simulink model "PMSMvelocityController"  (R2013b)
settings: Solver=FixedStepDiscrete  StartTime=0.0  StopTime=inf  RelTol=1e-3
values from neighbouring files (symbols this model uses):
  ctrlConst = struct    [applicationData.m]
  paramCurrentI = createParameter(      20000,      [0 25000],      DT_PRECISION_LO,      'Volt/Ampere',     'I gain parameter in Currrent Control PI Controller')    [applicationData.m]
  paramCurrentP = createParameter(     10,     [0 100],     DT_PRECISION_LO,     'Volt/Ampere',     'P gain parameter in Current Control PI Controller')    [applicationData.m]
  paramCurrentPIVoltageSat = createParameter(     0.9 * (ctrlConst.VoltageMax/2),     [0 (ctrlConst.VoltageMax/2)],     DT_PRECISION_LO,     'Volt',     'Maximum voltage command output from current controller')    [applicationData.m]
  paramVelocityI = createParameter(      0.275,      [0 2],      DT_PRECISION_LO,      'Ampere/(rad/sec)',     'I gain parameter in Velocity Control PI Controller')    [applicationData.m]
  paramVelocityP = createParameter(     0.2814,     [0 1],     DT_PRECISION_LO,     'Ampere/(rad/sec)',     'P gain parameter in Velocity Control PI Controller')    [applicationData.m]
  paramVelocityPICurrentSat = createParameter(     2,     [0 6],     DT_PRECISION_LO,     'Ampere',     'Maximum Current Command Output from Velocity Controller')    [applicationData.m]
libraries: simulink x11, libDataType x3, libAbcDqFixpt x2, libSinCosFixpt x1, libSinCosFixptC2000 x1, libSinCos x1
settings Model: SimulationMode=accelerator  Creator=mcorless  LastModifiedBy=rchladny
settings DataIOCC: SaveOutput=off  SaveTime=off
settings OptimizationCC: InlineParams=on  UseSpecifiedMinMax=on  ZeroExternalMemoryAtStartup=off  NoFixptDivByZeroProtection=on  EfficientFloat2IntCast=on  OptimizeModelRefInitCode=on  LifeSpan=1
settings DebuggingCC: InheritedTsInSrcMsg=none  ParameterPrecisionLossMsg=none  ModelReferenceSymbolNameMessage=none  StateNameClashWarn=warning
settings HardwareCC: ProdBitPerChar=16  ProdBitPerInt=16  ProdBitPerPointer=16  ProdLargestAtomicInteger=Integer  ProdIntDivRoundTo=Zero  ProdEndianess=LittleEndian  ProdWordSize=16  ProdHWDeviceType=Texas Instruments->C2000
settings ModelReferenceCC: ModelReferenceNumInstancesAllowed=Single
settings RTWCC: SystemTargetFile=ert.tlc  TemplateMakefile=ec_target.tmf  Description=Embedded Coder  GenerateReport=on  ProcessScript=ert_make_rtw_hook  IncludeHyperlinkInReport=on  LaunchReport=on  PortableWordSizes=on  GenerateTraceInfo=on  GenerateTraceReport=on  GenerateTraceReportSl=on  GenerateTraceReportSf=on  GenerateTraceReportEml=on  GenerateCodeMetricsReport=on  RTWCompilerOptimization=On
settings CodeAppCC: IgnoreCustomStorageClasses=off
settings ERTTargetCC: CodeReplacementLibrary=C89/C90 (ANSI)  GenerateSampleERTMain=on  IncludeMdlTerminateFcn=off  CombineSignalStateStructs=on  SuppressErrorStatus=on  ERTCustomFileTemplate=example_file_process.tlc  ERTFilePackagingFormat=Compact  SuppressUnreachableDefaultCases=on

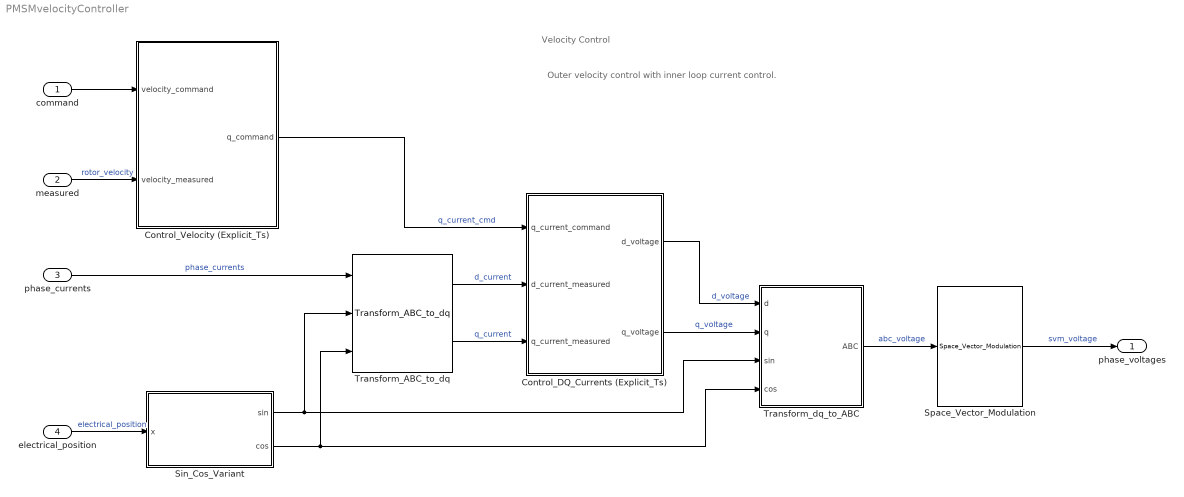
== system PMSMvelocityController ==
  note: Outer velocity control with inner loop current control.
  note: Velocity Control
  command : Inport  OutMin=-ctrlConst.VelocityMax  OutMax=ctrlConst.VelocityMax  OutDataTypeStr=DT_PRECISION_LO  PortDimensions=1  SampleTime=ctrlConst.TsControlLawPort  Interpolate=off
      settings: AttributesFormatString=-------------------\nMin = %<OutMin>\nMax = %<OutMax>
  measured : Inport  Port=2  OutMin=-ctrlConst.VelocityMax  OutMax=ctrlConst.VelocityMax  OutDataTypeStr=DT_PRECISION_LO  PortDimensions=1
      settings: AttributesFormatString=-------------------\nMin = %<OutMin>\nMax = %<OutMax>
  phase_currents : Inport  Port=3  OutMin=-ctrlConst.CurrentMax  OutMax=ctrlConst.CurrentMax  OutDataTypeStr=DT_PRECISION_LO  PortDimensions=2  Interpolate=off
      settings: AttributesFormatString=-------------------\nMin = %<OutMin>\nMax = %<OutMax>
  electrical_position : Inport  Port=4  OutMin=0  OutMax=2*pi  OutDataTypeStr=DT_PRECISION_LO  PortDimensions=1  Interpolate=off
      settings: AttributesFormatString=-------------------\nMin = %<OutMin>\nMax = %<OutMax>
  Control_DQ_Currents (Explicit_Ts) : Subsystem  Description=|  AncestorBlock=|  RTWFcnName=ControlCurrent
      Description=|
      | Linear Current Controllers
      | 
      | PID Blocks used for Control Design of Current Loop controllers.
      AncestorBlock=|
      | libControlCurrentFixpt/Control_DQ_Currents
      | (Explicit_Ts)
      settings: RTWFcnNameOpts=User specified
      mask Display: fprintf('Control DQ Currents\n(Quadrature = Input\nDirect = 0)')
  Control_Velocity (Explicit_Ts) : Subsystem  AncestorBlock=|
      | libControlVelocityFixpt/Control_Velocity
      | (Explicit_Ts)
      mask Display: fprintf('Control\nVelocity')
  Sin_Cos_Variant : Subsystem  Variant=on
  Space_Vector_Modulation : libAbcDqFixpt/Space_Vector_Modulation  SystemSampleTime=-1  VariantControl=SpaceVectorModulation_JB
  Transform_ABC_to_dq : libAbcDqFixpt/Transform_ABC_to_dq  SystemSampleTime=-1
  Transform_dq_to_ABC : Subsystem  AncestorBlock=libAbcDqFixpt/Transform_dq_to_ABC  TreatAsAtomicUnit=on  RTWFcnName=TransformDQToABCWithSVM
      settings: RTWFcnNameOpts=User specified
      mask Display: disp('Transform\nCoordinates\ndq to ABC')
  phase_voltages : Outport  PortDimensions=3
  wires:
  Sin_Cos_Variant/1(sin) -> Transform_ABC_to_dq/2, Transform_dq_to_ABC/3(sin)
  Sin_Cos_Variant/2(cos) -> Transform_dq_to_ABC/4(cos), Transform_ABC_to_dq/3
  Transform_dq_to_ABC/1(ABC) -> Space_Vector_Modulation/1  "abc_voltage"
  electrical_position/1 -> Sin_Cos_Variant/1(x)  "electrical_position"
  Space_Vector_Modulation/1 -> phase_voltages/1  "svm_voltage"
  Control_DQ_Currents (Explicit_Ts)/2(q_voltage) -> Transform_dq_to_ABC/2(q)  "q_voltage"
  Transform_ABC_to_dq/2 -> Control_DQ_Currents (Explicit_Ts)/3(q_current_measured)  "q_current"
  Transform_ABC_to_dq/1 -> Control_DQ_Currents (Explicit_Ts)/2(d_current_measured)  "d_current"
  phase_currents/1 -> Transform_ABC_to_dq/1  "phase_currents"
  Control_DQ_Currents (Explicit_Ts)/1(d_voltage) -> Transform_dq_to_ABC/1(d)  "d_voltage"
  measured/1 -> Control_Velocity (Explicit_Ts)/2(velocity_measured)  "rotor_velocity"
  command/1 -> Control_Velocity (Explicit_Ts)/1(velocity_command)
  Control_Velocity (Explicit_Ts)/1(q_command) -> Control_DQ_Currents (Explicit_Ts)/1(q_current_command)  "q_current_cmd"

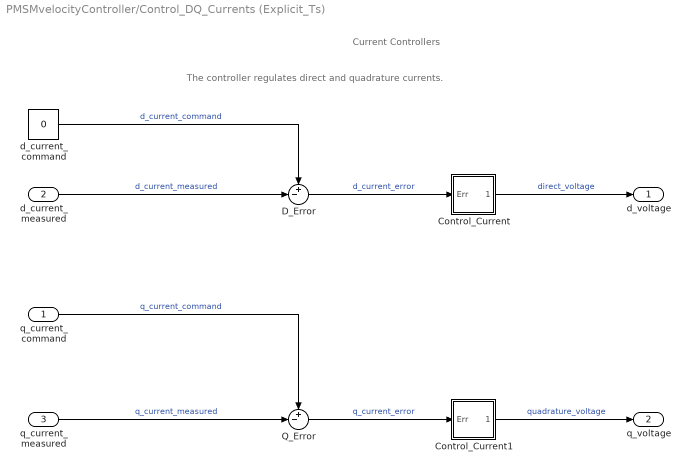
== system PMSMvelocityController/Control_DQ_Currents (Explicit_Ts) ==
  note: The controller regulates direct and quadrature currents.
  note: Current Controllers
  q_current_command : Inport  OutMin=-ctrlConst.CurrentMax  OutMax=ctrlConst.CurrentMax
      settings: AttributesFormatString=--------------------------------------\nMin = %<OutMin>\nMax = %<OutMax>
  d_current_measured : Inport  Port=2  OutMin=-ctrlConst.CurrentMax  OutMax=ctrlConst.CurrentMax  OutDataTypeStr=DT_PRECISION_LO
      settings: AttributesFormatString=--------------------------------------\nMin = %<OutMin>\nMax = %<OutMax>
  q_current_measured : Inport  Port=3  OutMin=-ctrlConst.CurrentMax  OutMax=ctrlConst.CurrentMax  OutDataTypeStr=DT_PRECISION_LO
      settings: AttributesFormatString=--------------------------------------\nMin = %<OutMin>\nMax = %<OutMax>
  Control_Current : Subsystem  TreatAsAtomicUnit=on
      mask Display:
      | disp('PI(z)')
      | port_label('input',1, '');
      | port_label('output',1, '');
  Control_Current1 : Subsystem  TreatAsAtomicUnit=on
      mask Display:
      | disp('PI(z)')
      | port_label('input',1, '');
      | port_label('output',1, '');
  D_Error : Sum  Inputs=+-|  OutMin=-ctrlConst.CurrentMax * 2  OutMax=ctrlConst.CurrentMax * 2  OutDataTypeStr=DT_PRECISION_LO
      settings: AttributesFormatString=--------------------------------------\nMin = %<OutMin>\nMax = %<OutMax>
  Q_Error : Sum  Inputs=+-|  OutMin=-ctrlConst.CurrentMax * 2  OutMax=ctrlConst.CurrentMax * 2  OutDataTypeStr=DT_PRECISION_LO
      settings: AttributesFormatString=--------------------------------------\nMin = %<OutMin>\nMax = %<OutMax>
  d_current_command : Constant  Value=0  OutDataTypeStr=Inherit: Inherit via back propagation
  d_voltage : Outport
  q_voltage : Outport  Port=2
  wires:
  Control_Current1/1(Out) -> q_voltage/1  "quadrature_voltage"
  Control_Current/1(Out) -> d_voltage/1  "direct_voltage"
  q_current_measured/1 -> Q_Error/2  "q_current_measured"
  d_current_measured/1 -> D_Error/2  "d_current_measured"
  Q_Error/1 -> Control_Current1/1(Err)  "q_current_error"
  D_Error/1 -> Control_Current/1(Err)  "d_current_error"
  q_current_command/1 -> Q_Error/1  "q_current_command"
  d_current_command/1 -> D_Error/1  "d_current_command"

== system PMSMvelocityController/Control_Velocity (Explicit_Ts) ==
  note: The controller regulates motor velocity using rotor velocity feedback compared to a commanded velocity.
      | The output of the controller is the quadrature-winding current command which is directly proportional to the electromagnetic torque of the motor.
      | Since the motor being controlled is a Permanent Magnet Synchronous Machine, the rotor flux linkage is fixed (determined by the magnets),
      | hence the commanded direct-winding current is always zero.
  note: Velocity Controller
  velocity_command : Inport  OutMin=-ctrlConst.VelocityMax  OutMax=ctrlConst.VelocityMax
      settings: AttributesFormatString=-----------------------------\nMin = %<OutMin>\nMax = %<OutMax>
  velocity_measured : Inport  Port=2  OutMin=-ctrlConst.VelocityMax  OutMax=ctrlConst.VelocityMax
      settings: AttributesFormatString=-----------------------------\nMin = %<OutMin>\nMax = %<OutMax>
  Error Sum : Sum  Inputs=+-|  OutMin=-2*ctrlConst.VelocityMax  OutMax=2*ctrlConst.VelocityMax  OutDataTypeStr=DT_PRECISION_LO
      settings: AttributesFormatString=-----------------------------\nMin = %<OutMin>\nMax = %<OutMax>
  Rotor_Velocity_Control : Subsystem
      mask Display:
      | disp('PI(z)')
      | port_label('input',1, '');
      | port_label('output',1, '');
  q_command : Outport  InitialOutput=0
  wires:
  velocity_measured/1 -> Error Sum/2
  Error Sum/1 -> Rotor_Velocity_Control/1(Err)  "velocity_error"
  velocity_command/1 -> Error Sum/1
  Rotor_Velocity_Control/1(Out) -> q_command/1  "q_current_cmd"

== system PMSMvelocityController/Sin_Cos_Variant ==
  note: 1) Only subsystems can be added as variant choices at this level
      | 2) Blocks cannot be connected at this level as connectivity is
      | automatically determined at simulation, based on the active variant
  x : Inport
  Sin_Cos_Fixpt : libSinCosFixpt/Sin_Cos_Fixpt  SystemSampleTime=-1  VariantControl=sinCosVariant==sinCosEnum.FixPt
  Sin_Cos_Fixpt_C2000_Block : libSinCosFixptC2000/Sin_Cos_Fixpt_C2000_Block  SystemSampleTime=-1  VariantControl=sinCosVariant==sinCosEnum.FixPtC2000
  Sin_Cos_Float : libSinCos/Sin_Cos_Float  SystemSampleTime=-1  VariantControl=sinCosVariant==sinCosEnum.Float
  sin : Outport
  cos : Outport  Port=2

== system PMSMvelocityController/Transform_dq_to_ABC ==
  note: Converts the two coordinate time invariant system (dq) to a three-phase time and speed dependent system (ABC).
  note: Transform Coordinates dq to ABC
  d : Inport
  q : Inport  Port=2
  sin : Inport  Port=3  OutMin=-1  OutMax=1
  cos : Inport  Port=4  OutMin=-1  OutMax=1
  Inverse_Clarke_Transform : Subsystem  VariantControl=INVERSE_CLARKE_TRANSFORM
  Inverse_Park_Transform : Subsystem
  ABC : Outport
  wires:
  sin/1 -> Inverse_Park_Transform/3(sin_coefficient)
  cos/1 -> Inverse_Park_Transform/4(cos_coefficient)
  q/1 -> Inverse_Park_Transform/2(quadrature_voltage)
  Inverse_Clarke_Transform/1(phase_voltages) -> ABC/1
  Inverse_Park_Transform/2(beta_voltage) -> Inverse_Clarke_Transform/2(beta_voltage)
  Inverse_Park_Transform/1(alpha_voltage) -> Inverse_Clarke_Transform/1(alpha_voltage)
  d/1 -> Inverse_Park_Transform/1(direct_voltage)

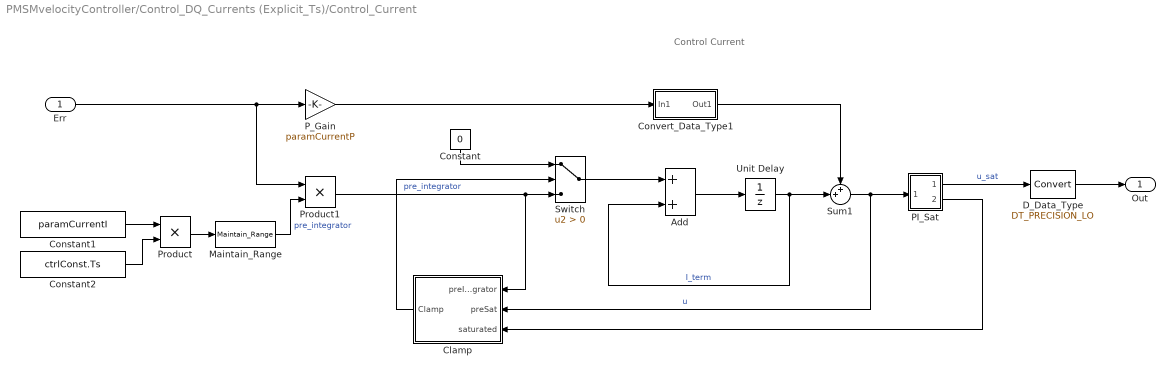
== system PMSMvelocityController/Control_DQ_Currents (Explicit_Ts)/Control_Current ==
  note: Control Current
  Err : Inport
  Add : Sum  OutMin=-ctrlConst.VoltageMax  OutMax=ctrlConst.VoltageMax  OutDataTypeStr=DT_PRECISION_HI  SaturateOnIntegerOverflow=on
      settings: AttributesFormatString=-----------------------------\nMin = %<OutMin>\nMax = %<OutMax>\nSat = %<SaturateOnIntegerOverflow>
  Clamp : Subsystem
  Constant : Constant  Value=0  OutDataTypeStr=Inherit: Inherit via back propagation  PreserveConstantTs=on
  Constant1 : Constant  Value=paramCurrentI  SampleTime=-1
  Constant2 : Constant  Value=ctrlConst.Ts  OutDataTypeStr=DT_PRECISION_LO  SampleTime=-1
  Convert_Data_Type1 : Subsystem
      mask Display: fprintf('Double\nRange')
  D_Data_Type : DataTypeConversion  OutMin=-ctrlConst.VoltageMax  OutMax=ctrlConst.VoltageMax  OutDataTypeStr=DT_PRECISION_LO
      settings: AttributesFormatString=--------------------------------------\nMin = %<OutMin>\nMax = %<OutMax>
  Maintain_Range : libDataType/Maintain_Range  SystemSampleTime=-1
  PI_Sat : Subsystem
      mask Display: plot([0.15 0.85],[.5 .5],[.5 .5],[0.05 0.95],0.15+0.7*[0 .25 .75 1],0.05+0.9*[.25 .25 .75 .75]);
  P_Gain : Gain  Gain=paramCurrentP  ParamDataTypeStr=Inherit: Inherit from 'Gain'
      settings: AttributesFormatString=-----------------------------\n%<Gain>
  Product : Product
  Product1 : Product
  Sum1 : Sum  Inputs=++|  OutDataTypeStr=Inherit: Inherit via back propagation
  Switch : Switch  Criteria=u2 > Threshold  InputSameDT=on
  Unit Delay : UnitDelay  SampleTime=-1
  Out : Outport
  wires:
  Maintain_Range/1 -> Product1/2  "pre_integrator"
  Product/1 -> Maintain_Range/1
  Constant2/1 -> Product/2
  Constant1/1 -> Product/1
  Convert_Data_Type1/1(Out1) -> Sum1/1
  PI_Sat/2(saturated) -> Clamp/3(saturated)
  Add/1 -> Unit Delay/1
  Switch/1 -> Add/1
  Unit Delay/1 -> Sum1/2, Add/2  "I_term"
  D_Data_Type/1 -> Out/1
  P_Gain/1 -> Convert_Data_Type1/1(In1)
  Sum1/1 -> PI_Sat/1(In1), Clamp/2(preSat)  "u"
  Err/1 -> Product1/1, P_Gain/1
  PI_Sat/1(Out1) -> D_Data_Type/1  "u_sat"
  Constant/1 -> Switch/1
  Clamp/1(Clamp) -> Switch/2
  Product1/1 -> Switch/3, Clamp/1(preIntegrator)  "pre_integrator"

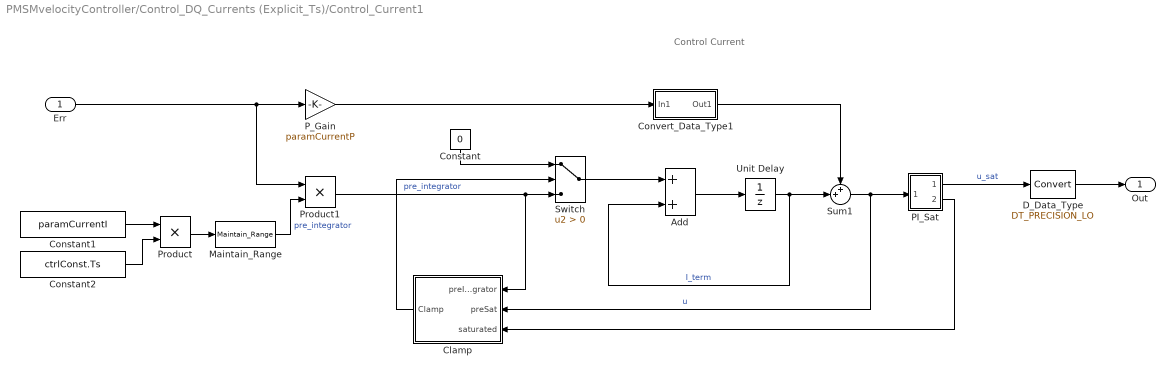
== system PMSMvelocityController/Control_DQ_Currents (Explicit_Ts)/Control_Current1 ==
  note: Control Current
  Err : Inport
  Add : Sum  OutMin=-ctrlConst.VoltageMax  OutMax=ctrlConst.VoltageMax  OutDataTypeStr=DT_PRECISION_HI  SaturateOnIntegerOverflow=on
      settings: AttributesFormatString=-----------------------------\nMin = %<OutMin>\nMax = %<OutMax>\nSat = %<SaturateOnIntegerOverflow>
  Clamp : Subsystem
  Constant : Constant  Value=0  OutDataTypeStr=Inherit: Inherit via back propagation  PreserveConstantTs=on
  Constant1 : Constant  Value=paramCurrentI  SampleTime=-1
  Constant2 : Constant  Value=ctrlConst.Ts  OutDataTypeStr=DT_PRECISION_LO  SampleTime=-1
  Convert_Data_Type1 : Subsystem
      mask Display: fprintf('Double\nRange')
  D_Data_Type : DataTypeConversion  OutMin=-ctrlConst.VoltageMax  OutMax=ctrlConst.VoltageMax  OutDataTypeStr=DT_PRECISION_LO
      settings: AttributesFormatString=--------------------------------------\nMin = %<OutMin>\nMax = %<OutMax>
  Maintain_Range : libDataType/Maintain_Range  SystemSampleTime=-1
  PI_Sat : Subsystem
      mask Display: plot([0.15 0.85],[.5 .5],[.5 .5],[0.05 0.95],0.15+0.7*[0 .25 .75 1],0.05+0.9*[.25 .25 .75 .75]);
  P_Gain : Gain  Gain=paramCurrentP  ParamDataTypeStr=Inherit: Inherit from 'Gain'
      settings: AttributesFormatString=-----------------------------\n%<Gain>
  Product : Product
  Product1 : Product
  Sum1 : Sum  Inputs=++|  OutDataTypeStr=Inherit: Inherit via back propagation
  Switch : Switch  Criteria=u2 > Threshold  InputSameDT=on
  Unit Delay : UnitDelay  SampleTime=-1
  Out : Outport
  wires:
  Product1/1 -> Clamp/1(preIntegrator), Switch/3  "pre_integrator"
  Clamp/1(Clamp) -> Switch/2
  Constant/1 -> Switch/1
  PI_Sat/1(Out1) -> D_Data_Type/1  "u_sat"
  Err/1 -> P_Gain/1, Product1/1
  Sum1/1 -> Clamp/2(preSat), PI_Sat/1(In1)  "u"
  P_Gain/1 -> Convert_Data_Type1/1(In1)
  D_Data_Type/1 -> Out/1
  Unit Delay/1 -> Add/2, Sum1/2  "I_term"
  Switch/1 -> Add/1
  Add/1 -> Unit Delay/1
  Convert_Data_Type1/1(Out1) -> Sum1/1
  Constant1/1 -> Product/1
  Constant2/1 -> Product/2
  Product/1 -> Maintain_Range/1
  Maintain_Range/1 -> Product1/2  "pre_integrator"
  PI_Sat/2(saturated) -> Clamp/3(saturated)

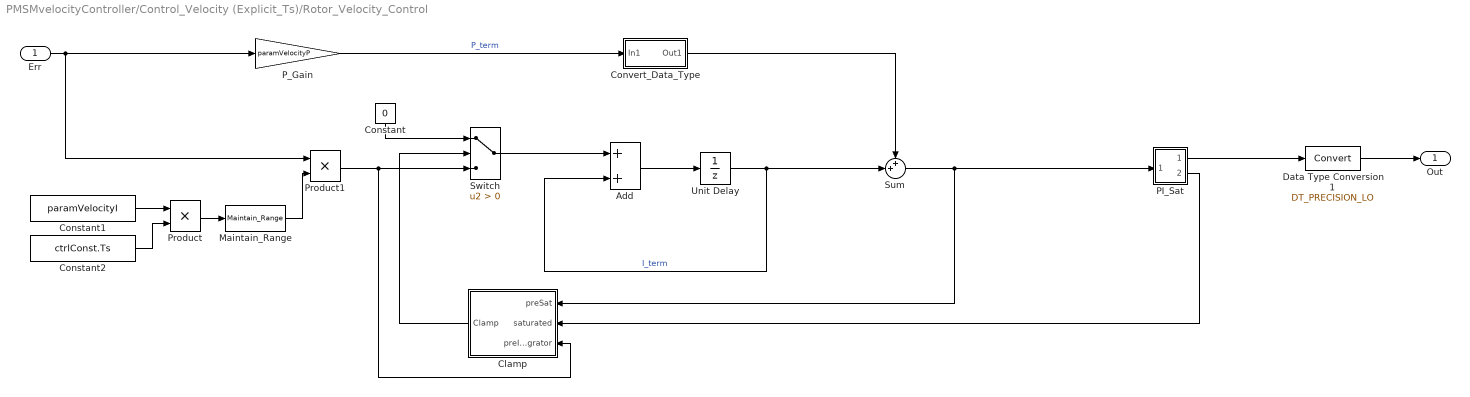
== system PMSMvelocityController/Control_Velocity (Explicit_Ts)/Rotor_Velocity_Control ==
  Err : Inport
  Add : Sum  OutMin=-ctrlConst.CurrentMax*2  OutMax=ctrlConst.CurrentMax*2  OutDataTypeStr=DT_PRECISION_HI  SaturateOnIntegerOverflow=on
      settings: AttributesFormatString=-----------------------------\nMin = %<OutMin>\nMax = %<OutMax>\nSat = %<SaturateOnIntegerOverflow>
  Clamp : Subsystem
  Constant : Constant  Value=0  OutDataTypeStr=Inherit: Inherit via back propagation  PreserveConstantTs=on
  Constant1 : Constant  Value=paramVelocityI  SampleTime=-1
  Constant2 : Constant  Value=ctrlConst.Ts  OutDataTypeStr=DT_PRECISION_LO  SampleTime=-1
  Convert_Data_Type : Subsystem
      mask Display: fprintf('Double\nRange')
  Data Type Conversion1 : DataTypeConversion  OutMin=-ctrlConst.CurrentMax  OutMax=ctrlConst.CurrentMax  OutDataTypeStr=DT_PRECISION_LO
      settings: AttributesFormatString=-----------------------------\nMin = %<OutMin>\nMax = %<OutMax>
  Maintain_Range : libDataType/Maintain_Range  SystemSampleTime=-1
  PI_Sat : Subsystem
      mask Display: plot([0.15 0.85],[.5 .5],[.5 .5],[0.05 0.95],0.15+0.7*[0 .25 .75 1],0.05+0.9*[.25 .25 .75 .75]);
  P_Gain : Gain  Gain=paramVelocityP  ParamDataTypeStr=Inherit: Inherit from 'Gain'
      settings: AttributesFormatString=-----------------------------\n%<Gain>
  Product : Product
  Product1 : Product
  Sum : Sum  Inputs=++|
  Switch : Switch  Criteria=u2 > Threshold  InputSameDT=on
  Unit Delay : UnitDelay  SampleTime=-1
  Out : Outport
  wires:
  Convert_Data_Type/1(Out1) -> Sum/1
  Data Type Conversion1/1 -> Out/1
  PI_Sat/1(Out1) -> Data Type Conversion1/1
  Switch/1 -> Add/1
  PI_Sat/2(saturated) -> Clamp/2(saturated)
  Err/1 -> Product1/1, P_Gain/1
  P_Gain/1 -> Convert_Data_Type/1(In1)  "P_term"
  Add/1 -> Unit Delay/1
  Unit Delay/1 -> Add/2, Sum/2  "I_term"
  Constant/1 -> Switch/1
  Clamp/1(Clamp) -> Switch/2
  Product1/1 -> Clamp/3(preIntegrator), Switch/3
  Constant1/1 -> Product/1
  Constant2/1 -> Product/2
  Product/1 -> Maintain_Range/1
  Maintain_Range/1 -> Product1/2
  Sum/1 -> PI_Sat/1(In1), Clamp/1(preSat)

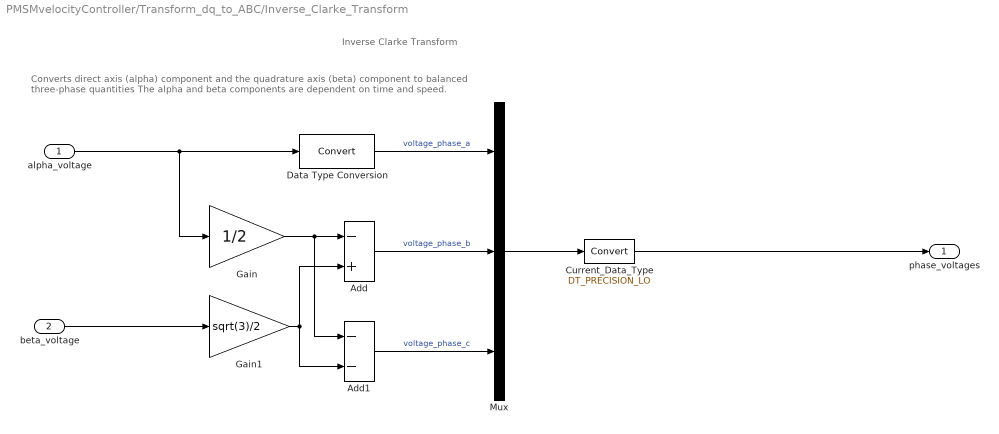
== system PMSMvelocityController/Transform_dq_to_ABC/Inverse_Clarke_Transform ==
  note: Converts direct axis (alpha) component and the quadrature axis (beta) component to balanced three-phase quantities
      | The alpha and beta components are dependent on time and speed.
  note: Inverse Clarke Transform
  alpha_voltage : Inport
  beta_voltage : Inport  Port=2
  Add : Sum  Inputs=-+  OutDataTypeStr=Inherit: Same as first input
  Add1 : Sum  Inputs=--  OutDataTypeStr=Inherit: Same as first input
  Current_Data_Type : DataTypeConversion  OutMin=-ctrlConst.VoltageMax / 2  OutMax=ctrlConst.VoltageMax /2  OutDataTypeStr=DT_PRECISION_LO  SaturateOnIntegerOverflow=on
      settings: AttributesFormatString=--------------------------------------\nSaturate = %<SaturateOnIntegerOverflow>\nMin = %<OutMin>\nMax = %<OutMax>
  Data Type Conversion : DataTypeConversion
  Gain : Gain  Gain=1/2  ParamMax=1/2 + sqrt(3)/2  ParamDataTypeStr=DT_PRECISION_LO
  Gain1 : Gain  Gain=sqrt(3)/2  ParamMax=1/2 + sqrt(3)/2  ParamDataTypeStr=DT_PRECISION_LO
  Mux : Mux  Inputs=3
  phase_voltages : Outport
  wires:
  Current_Data_Type/1 -> phase_voltages/1
  Data Type Conversion/1 -> Mux/1  "voltage_phase_a"
  alpha_voltage/1 -> Data Type Conversion/1, Gain/1
  beta_voltage/1 -> Gain1/1
  Add1/1 -> Mux/3  "voltage_phase_c"
  Add/1 -> Mux/2  "voltage_phase_b"
  Gain1/1 -> Add/2, Add1/2
  Gain/1 -> Add/1, Add1/1
  Mux/1 -> Current_Data_Type/1

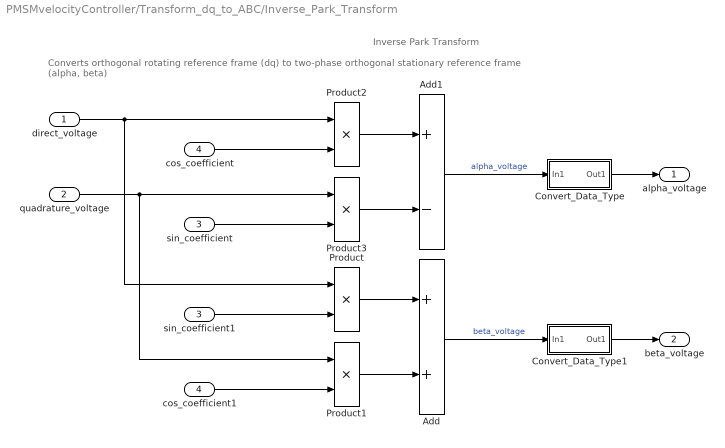
== system PMSMvelocityController/Transform_dq_to_ABC/Inverse_Park_Transform ==
  note: Converts orthogonal rotating reference frame (dq) to two-phase orthogonal stationary reference frame (alpha, beta)
  note: Inverse Park Transform
  direct_voltage : Inport
  quadrature_voltage : Inport  Port=2
  sin_coefficient : Inport  Port=3
  cos_coefficient : Inport  Port=4
  Add : Sum  InputSameDT=on  OutDataTypeStr=Inherit: Same as first input
  Add1 : Sum  Inputs=+-  InputSameDT=on  OutDataTypeStr=Inherit: Same as first input
  Convert_Data_Type : Subsystem
      mask Display: fprintf('Maintain\nRange')
  Convert_Data_Type1 : Subsystem
      mask Display: fprintf('Maintain\nRange')
  Product{,1..3} (4 alike) : Product  RndMeth=Simplest
  cos_coefficient1 : InportShadow  Port=4
  sin_coefficient1 : InportShadow  Port=3
  alpha_voltage : Outport
  beta_voltage : Outport  Port=2
  wires:
  cos_coefficient/1 -> Product2/2
  sin_coefficient1/1 -> Product/2
  quadrature_voltage/1 -> Product1/1, Product3/1
  direct_voltage/1 -> Product/1, Product2/1
  sin_coefficient/1 -> Product3/2
  cos_coefficient1/1 -> Product1/2
  Product3/1 -> Add1/2
  Product2/1 -> Add1/1
  Product1/1 -> Add/2
  Product/1 -> Add/1
  Add1/1 -> Convert_Data_Type/1(In1)  "alpha_voltage"
  Convert_Data_Type/1(Out1) -> alpha_voltage/1
  Add/1 -> Convert_Data_Type1/1(In1)  "beta_voltage"
  Convert_Data_Type1/1(Out1) -> beta_voltage/1

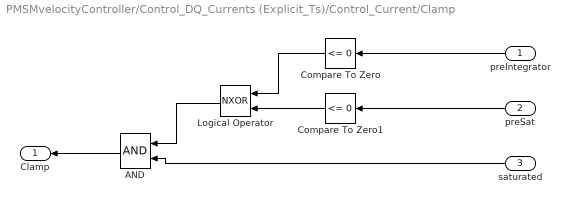
== system PMSMvelocityController/Control_DQ_Currents (Explicit_Ts)/Control_Current/Clamp ==
  preIntegrator : Inport
  preSat : Inport  Port=2
  saturated : Inport  Port=3
  AND : Logic  OutDataTypeStr=boolean
  Compare To Zero : simulink/Logic and Bit Operations/Compare To Zero  relop=<=  OutDataTypeStr=boolean
  Compare To Zero1 : simulink/Logic and Bit Operations/Compare To Zero  relop=<=  OutDataTypeStr=boolean
  Logical Operator : Logic  Operator=NXOR  AllPortsSameDT=off  OutDataTypeStr=boolean
  Clamp : Outport
  wires:
  AND/1 -> Clamp/1
  saturated/1 -> AND/2
  preIntegrator/1 -> Compare To Zero/1
  preSat/1 -> Compare To Zero1/1
  Logical Operator/1 -> AND/1
  Compare To Zero/1 -> Logical Operator/1
  Compare To Zero1/1 -> Logical Operator/2

== system PMSMvelocityController/Control_DQ_Currents (Explicit_Ts)/Control_Current/Convert_Data_Type1 ==
  In1 : Inport
  Data Type Conversion : DataTypeConversion  Priority=27
  Data Type Propagation : simulink/Signal Attributes/Data Type Propagation  Priority=24  PropDataType=fixdt(1, 16)  IfRefDouble=double  IfRefSingle=single  IsSigned=IsSigned1  NumBitsBase=NumBits1  NumBitsMult=1  NumBitsAdd=0  NumBitsAllowFinal=1:128  PropScaling=2^-10  ValuesUsedBestPrec=[5 -7]  SlopeBase=Slope1  SlopeMult=2  SlopeAdd=0  BiasBase=Bias1  BiasMult=1  BiasAdd=0
      settings: AttributesFormatString=-------------------------------\nDT = %<PropDataType>
  Out1 : Outport
  wires:
  In1/1 -> Data Type Propagation/2, Data Type Propagation/1, Data Type Conversion/1
  Data Type Conversion/1 -> Out1/1, Data Type Propagation/3

== system PMSMvelocityController/Control_DQ_Currents (Explicit_Ts)/Control_Current/PI_Sat ==
  In1 : Inport
  Dynamic Saturation : Subsystem
      mask Display: plot([0.15 0.85],[.5 .5],[.5 .5],[0.05 0.95],0.15+0.7*[0 .25 .75 1],0.05+0.9*[.25 .25 .75 .75]);
  PI_Sat : Constant  Value=paramCurrentPIVoltageSat  PreserveConstantTs=on
  Unary Minus : UnaryMinus
  Out1 : Outport
  saturated : Outport  Port=2
  wires:
  Dynamic Saturation/2(sat_mode) -> saturated/1
  Dynamic Saturation/1(y) -> Out1/1
  Unary Minus/1 -> Dynamic Saturation/3(lo)
  PI_Sat/1 -> Dynamic Saturation/1(up), Unary Minus/1
  In1/1 -> Dynamic Saturation/2(u)

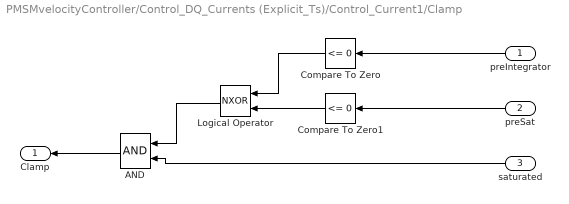
== system PMSMvelocityController/Control_DQ_Currents (Explicit_Ts)/Control_Current1/Clamp ==
  preIntegrator : Inport
  preSat : Inport  Port=2
  saturated : Inport  Port=3
  AND : Logic  OutDataTypeStr=boolean
  Compare To Zero : simulink/Logic and Bit Operations/Compare To Zero  relop=<=  OutDataTypeStr=boolean
  Compare To Zero1 : simulink/Logic and Bit Operations/Compare To Zero  relop=<=  OutDataTypeStr=boolean
  Logical Operator : Logic  Operator=NXOR  AllPortsSameDT=off  OutDataTypeStr=boolean
  Clamp : Outport
  wires:
  Compare To Zero1/1 -> Logical Operator/2
  Compare To Zero/1 -> Logical Operator/1
  Logical Operator/1 -> AND/1
  preSat/1 -> Compare To Zero1/1
  preIntegrator/1 -> Compare To Zero/1
  saturated/1 -> AND/2
  AND/1 -> Clamp/1

== system PMSMvelocityController/Control_DQ_Currents (Explicit_Ts)/Control_Current1/Convert_Data_Type1 ==
  In1 : Inport
  Data Type Conversion : DataTypeConversion  Priority=27
  Data Type Propagation : simulink/Signal Attributes/Data Type Propagation  Priority=24  PropDataType=fixdt(1, 16)  IfRefDouble=double  IfRefSingle=single  IsSigned=IsSigned1  NumBitsBase=NumBits1  NumBitsMult=1  NumBitsAdd=0  NumBitsAllowFinal=1:128  PropScaling=2^-10  ValuesUsedBestPrec=[5 -7]  SlopeBase=Slope1  SlopeMult=2  SlopeAdd=0  BiasBase=Bias1  BiasMult=1  BiasAdd=0
      settings: AttributesFormatString=-------------------------------\nDT = %<PropDataType>
  Out1 : Outport
  wires:
  Data Type Conversion/1 -> Data Type Propagation/3, Out1/1
  In1/1 -> Data Type Conversion/1, Data Type Propagation/1, Data Type Propagation/2

== system PMSMvelocityController/Control_DQ_Currents (Explicit_Ts)/Control_Current1/PI_Sat ==
  In1 : Inport
  Dynamic Saturation : Subsystem
      mask Display: plot([0.15 0.85],[.5 .5],[.5 .5],[0.05 0.95],0.15+0.7*[0 .25 .75 1],0.05+0.9*[.25 .25 .75 .75]);
  PI_Sat : Constant  Value=paramCurrentPIVoltageSat  PreserveConstantTs=on
  Unary Minus : UnaryMinus
  Out1 : Outport
  saturated : Outport  Port=2
  wires:
  In1/1 -> Dynamic Saturation/2(u)
  PI_Sat/1 -> Unary Minus/1, Dynamic Saturation/1(up)
  Unary Minus/1 -> Dynamic Saturation/3(lo)
  Dynamic Saturation/1(y) -> Out1/1
  Dynamic Saturation/2(sat_mode) -> saturated/1

== system PMSMvelocityController/Control_Velocity (Explicit_Ts)/Rotor_Velocity_Control/Clamp ==
  preSat : Inport
  saturated : Inport  Port=2
  preIntegrator : Inport  Port=3
  AND : Logic  OutDataTypeStr=boolean
  Compare To Zero : simulink/Logic and Bit Operations/Compare To Zero  relop=<=  OutDataTypeStr=boolean
  Compare To Zero1 : simulink/Logic and Bit Operations/Compare To Zero  relop=<=  OutDataTypeStr=boolean
  Logical Operator : Logic  Operator=NXOR  AllPortsSameDT=off  OutDataTypeStr=boolean
  Clamp : Outport
  wires:
  AND/1 -> Clamp/1
  saturated/1 -> AND/2
  preIntegrator/1 -> Compare To Zero/1
  preSat/1 -> Compare To Zero1/1
  Logical Operator/1 -> AND/1
  Compare To Zero/1 -> Logical Operator/1
  Compare To Zero1/1 -> Logical Operator/2

== system PMSMvelocityController/Control_Velocity (Explicit_Ts)/Rotor_Velocity_Control/Convert_Data_Type ==
  In1 : Inport
  Data Type Conversion : DataTypeConversion  Priority=27
  Data Type Propagation : simulink/Signal Attributes/Data Type Propagation  Priority=24  PropDataType=fixdt(1, 16)  IfRefDouble=double  IfRefSingle=single  IsSigned=IsSigned1  NumBitsBase=NumBits1  NumBitsMult=1  NumBitsAdd=0  NumBitsAllowFinal=1:128  PropScaling=2^-10  ValuesUsedBestPrec=[5 -7]  SlopeBase=Slope1  SlopeMult=2  SlopeAdd=0  BiasBase=Bias1  BiasMult=1  BiasAdd=0
      settings: AttributesFormatString=-------------------------------\nDT = %<PropDataType>
  Out1 : Outport
  wires:
  In1/1 -> Data Type Propagation/2, Data Type Propagation/1, Data Type Conversion/1
  Data Type Conversion/1 -> Out1/1, Data Type Propagation/3

== system PMSMvelocityController/Control_Velocity (Explicit_Ts)/Rotor_Velocity_Control/PI_Sat ==
  In1 : Inport
  Dynamic Saturation : Subsystem
      mask Display: plot([0.15 0.85],[.5 .5],[.5 .5],[0.05 0.95],0.15+0.7*[0 .25 .75 1],0.05+0.9*[.25 .25 .75 .75]);
  PI_Sat : Constant  Value=paramVelocityPICurrentSat  PreserveConstantTs=on
  Unary Minus : UnaryMinus
  Out1 : Outport
  saturated : Outport  Port=2
  wires:
  Dynamic Saturation/2(sat_mode) -> saturated/1
  Dynamic Saturation/1(y) -> Out1/1
  Unary Minus/1 -> Dynamic Saturation/3(lo)
  PI_Sat/1 -> Dynamic Saturation/1(up), Unary Minus/1
  In1/1 -> Dynamic Saturation/2(u)

== system PMSMvelocityController/Transform_dq_to_ABC/Inverse_Park_Transform/Convert_Data_Type ==
  In1 : Inport
  Data Type Conversion : DataTypeConversion
  Data Type Propagation : simulink/Signal Attributes/Data Type Propagation  PropDataTypeMode=Specify via dialog  PropDataType=DT_PRECISION_LO  IfRefDouble=double  IfRefSingle=single  IsSigned=IsSigned1  NumBitsBase=NumBits1  NumBitsMult=0  NumBitsAdd=0  NumBitsAllowFinal=1:128  PropScaling=2^-10  ValuesUsedBestPrec=[5 -7]  SlopeBase=PosRange1  SlopeMult=1  SlopeAdd=0  BiasBase=Bias1  BiasMult=1  BiasAdd=0
      settings: AttributesFormatString=-------------------------------\nDT = %<PropDataType>
  Out1 : Outport
  wires:
  Data Type Conversion/1 -> Data Type Propagation/3, Out1/1
  In1/1 -> Data Type Conversion/1, Data Type Propagation/1, Data Type Propagation/2

== system PMSMvelocityController/Transform_dq_to_ABC/Inverse_Park_Transform/Convert_Data_Type1 ==
  In1 : Inport
  Data Type Conversion : DataTypeConversion
  Data Type Propagation : simulink/Signal Attributes/Data Type Propagation  PropDataTypeMode=Specify via dialog  PropDataType=DT_PRECISION_LO  IfRefDouble=double  IfRefSingle=single  IsSigned=IsSigned1  NumBitsBase=NumBits1  NumBitsMult=0  NumBitsAdd=0  NumBitsAllowFinal=1:128  PropScaling=2^-10  ValuesUsedBestPrec=[5 -7]  SlopeBase=PosRange1  SlopeMult=1  SlopeAdd=0  BiasBase=Bias1  BiasMult=1  BiasAdd=0
      settings: AttributesFormatString=-------------------------------\nDT = %<PropDataType>
  Out1 : Outport
  wires:
  Data Type Conversion/1 -> Data Type Propagation/3, Out1/1
  In1/1 -> Data Type Conversion/1, Data Type Propagation/1, Data Type Propagation/2

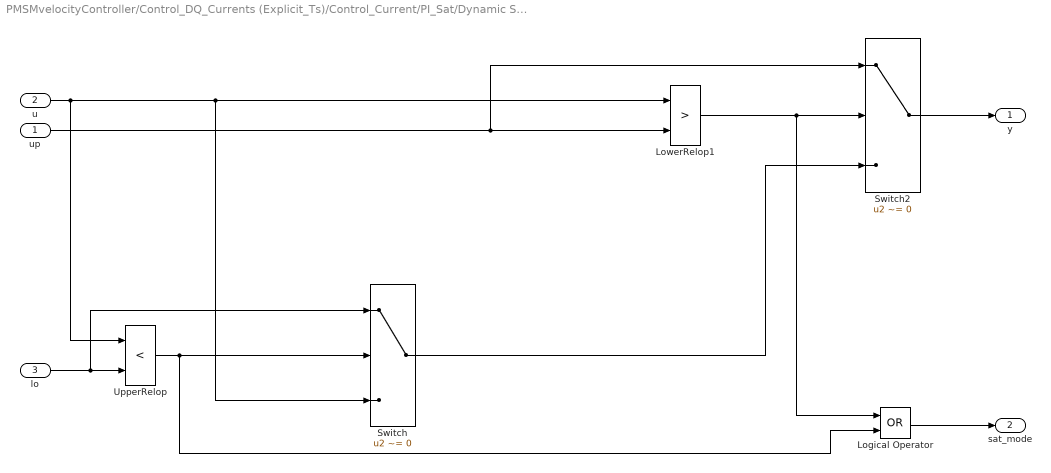
== system PMSMvelocityController/Control_DQ_Currents (Explicit_Ts)/Control_Current/PI_Sat/Dynamic Saturation ==
  up : Inport
  u : Inport  Port=2
  lo : Inport  Port=3
  Logical Operator : Logic  Operator=OR  AllPortsSameDT=off  OutDataTypeStr=boolean
  LowerRelop1 : RelationalOperator  DisableCoverage=on  Operator=>  OutDataTypeStr=boolean
  Switch : Switch  Criteria=u2 ~= 0  ZeroCross=off
  Switch2 : Switch  Criteria=u2 ~= 0  ZeroCross=off
  UpperRelop : RelationalOperator  DisableCoverage=on  Operator=<  OutDataTypeStr=boolean
  y : Outport
  sat_mode : Outport  Port=2
  wires:
  Logical Operator/1 -> sat_mode/1
  up/1 -> Switch2/1, LowerRelop1/2
  u/1 -> LowerRelop1/1, Switch/3, UpperRelop/1
  lo/1 -> Switch/1, UpperRelop/2
  Switch/1 -> Switch2/3
  Switch2/1 -> y/1
  LowerRelop1/1 -> Switch2/2, Logical Operator/1
  UpperRelop/1 -> Switch/2, Logical Operator/2

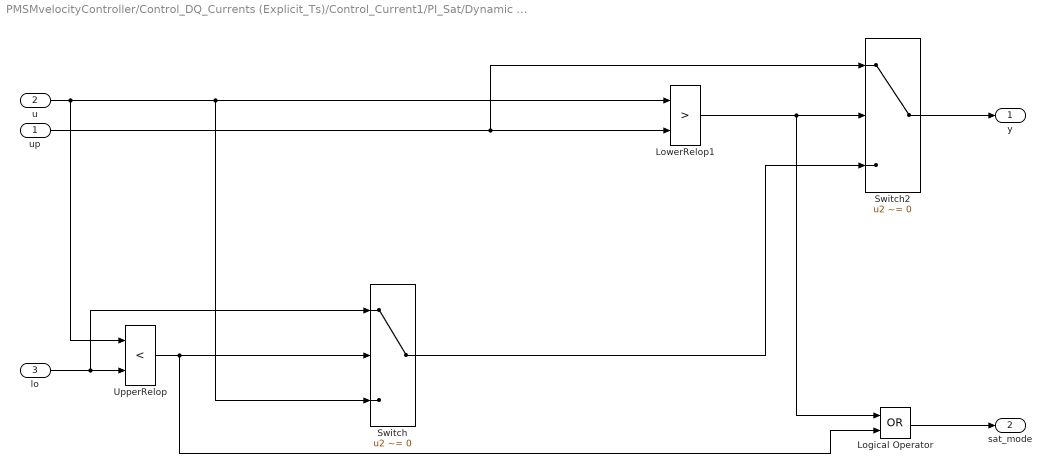
== system PMSMvelocityController/Control_DQ_Currents (Explicit_Ts)/Control_Current1/PI_Sat/Dynamic Saturation ==
  up : Inport
  u : Inport  Port=2
  lo : Inport  Port=3
  Logical Operator : Logic  Operator=OR  AllPortsSameDT=off  OutDataTypeStr=boolean
  LowerRelop1 : RelationalOperator  DisableCoverage=on  Operator=>  OutDataTypeStr=boolean
  Switch : Switch  Criteria=u2 ~= 0  ZeroCross=off
  Switch2 : Switch  Criteria=u2 ~= 0  ZeroCross=off
  UpperRelop : RelationalOperator  DisableCoverage=on  Operator=<  OutDataTypeStr=boolean
  y : Outport
  sat_mode : Outport  Port=2
  wires:
  UpperRelop/1 -> Logical Operator/2, Switch/2
  LowerRelop1/1 -> Logical Operator/1, Switch2/2
  Switch2/1 -> y/1
  Switch/1 -> Switch2/3
  lo/1 -> UpperRelop/2, Switch/1
  u/1 -> UpperRelop/1, Switch/3, LowerRelop1/1
  up/1 -> LowerRelop1/2, Switch2/1
  Logical Operator/1 -> sat_mode/1

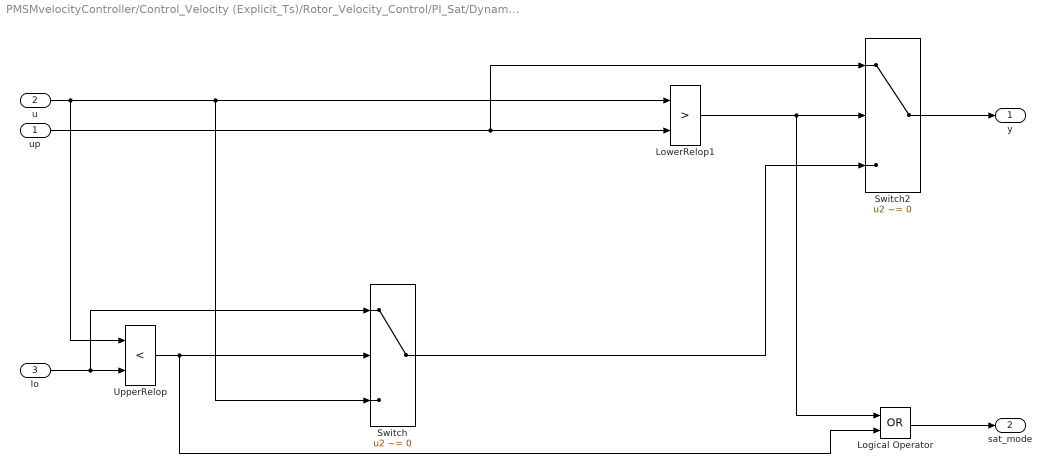
== system PMSMvelocityController/Control_Velocity (Explicit_Ts)/Rotor_Velocity_Control/PI_Sat/Dynamic Saturation ==
  up : Inport
  u : Inport  Port=2
  lo : Inport  Port=3
  Logical Operator : Logic  Operator=OR  AllPortsSameDT=off  OutDataTypeStr=boolean
  LowerRelop1 : RelationalOperator  DisableCoverage=on  Operator=>  OutDataTypeStr=boolean
  Switch : Switch  Criteria=u2 ~= 0  ZeroCross=off
  Switch2 : Switch  Criteria=u2 ~= 0  ZeroCross=off
  UpperRelop : RelationalOperator  DisableCoverage=on  Operator=<  OutDataTypeStr=boolean
  y : Outport
  sat_mode : Outport  Port=2
  wires:
  Logical Operator/1 -> sat_mode/1
  up/1 -> Switch2/1, LowerRelop1/2
  u/1 -> LowerRelop1/1, Switch/3, UpperRelop/1
  lo/1 -> Switch/1, UpperRelop/2
  Switch/1 -> Switch2/3
  Switch2/1 -> y/1
  LowerRelop1/1 -> Switch2/2, Logical Operator/1
  UpperRelop/1 -> Switch/2, Logical Operator/2
